simulink model "UARTReadLine1"  (R2017b)
settings: Solver=FixedStepDiscrete  StartTime=0.0  StopTime=10.0  FixedStep=1e-3  RelTol=1e-3
libraries: mbed_lib x3
settings Model: Creator=oh  LastModifiedBy=oh
settings DataIOCC: LimitDataPoints=on  SaveFormat=Array
settings OptimizationCC: LifeSpan=1
settings DebuggingCC: SFUnexpectedBacktrackingDiag=warning  SFNoUnconditionalDefaultTransitionDiag=warning  SFExecutionAtInitializationDiag=none
settings HardwareCC: ProdBitPerPointer=32  ProdBitPerSizeT=32  ProdBitPerPtrDiffT=32  ProdLargestAtomicInteger=Long  ProdLargestAtomicFloat=Double  ProdIntDivRoundTo=Undefined  ProdWordSize=32  ProdHWDeviceType=ARM Compatible->ARM Cortex
settings ModelReferenceCC: PropagateSignalLabelsOutOfModel=off
settings SFSimCC: MATLABDynamicMemAlloc=off
settings RTWCC: SystemTargetFile=mbed.tlc  TemplateMakefile=mbed.tmf  Description=Mbed Target (Embedded Target)  TargetLang=C++
settings CodeAppCC: IgnoreCustomStorageClasses=off  StateflowObjectComments=on
settings STFCustomTargetCC: TargetLibSuffix=.a  GenerateSampleERTMain=on  CombineOutputUpdateFcns=on  ERTCustomFileBanners=on  SupportContinuousTime=off  SupportNonInlinedSFcns=off  RemoveResetFunc=on  SupportVariableSizeSignals=on  MATLABClassNameForMDSCustomization=Simulink.SoftwareTarget.ERTCustomization  ModelStepFunctionPrototypeControlCompliant=on  GRTInterface=off  SystemTargetFile=mbed.tlc
settings ERTTargetCC: MultiwordLength=2048  GenerateSampleERTMain=on  ParMdlRefBuildCompliant=off  CompOptLevelCompliant=off  ConcurrentExecutionCompliant=off  SupportVariableSizeSignals=on  CPPClassGenCompliant=off  UseToolchainInfoCompliant=off  ERTCustomFileTemplate=mbed_file_process.tlc  ConvertIfToSwitch=off  SuppressUnreachableDefaultCases=off
settings ConfigComp: CovMetricSettings=dw  CovHtmlReporting=on  CovSaveCumulativeToWorkspaceVar=on  CovSaveSingleToWorkspaceVar=on  CovExternalEMLEnable=off

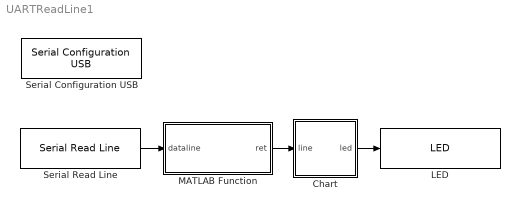
== system UARTReadLine1 ==
  Chart : Stateflow chart  TreatAsAtomicUnit=on
  LED : mbed_lib/GPIO/LED  nLED=1  SampleTime=-1
      settings: SourceProductName=Mbed Target
  MATLAB Function : MATLAB Function  TreatAsAtomicUnit=on
  Serial Configuration USB : mbed_lib/Serial/UART/Serial Configuration USB  Priority=0  BaudRate=9600
      settings: AttributesFormatString=%<Priority>=10  SourceProductName=Mbed Target
  Serial Read Line : mbed_lib/Serial/UART/Serial Read Line  SerialPort=USB  NumDataPort=off  NewDataPort=off  BufferSize=5  SampleTime=0.5
      settings: SourceProductName=Mbed Target
  wires:
  Chart/1(led) -> LED/1
  MATLAB Function/1(ret) -> Chart/1(line)
  Serial Read Line/1 -> MATLAB Function/1(dataline)

== matlab function UARTReadLine1/MATLAB Function ==
  data: ret output; dataline input
function ret = strmulticompare(dataline)

commands = {'on', 'off'};

ret = uint8(0);

for i=1:size(commands,2)
    ok=uint8(1);
    for j=1:size(commands{i},2)
        if commands{i}(j)~=dataline(j)
            ok=uint8(0);
            break;
        end
    end
    if ok==uint8(1)
      ret = uint8(i);
      return;
    end
end

== stateflow chart UARTReadLine1/Chart ==
  state start
  (default) -> start
  start -> start [order 1] : [line==uint8(1)]{led=1;}
  start -> start [order 2] : [line==uint8(2)]{led=0;}
  data: line input; led output uint8
